simulink model "subsystem_enable_triggered"  (R2022b)
settings: Solver=VariableStepAuto  StartTime=0.0  StopTime=0.1  FixedStep=0.01  MaxStep=1e-3  RelTol=1e-3
settings Model: Creator=Dell  LastModifiedBy=Dell
settings OptimizationCC: DefaultParameterBehavior=Inlined  UseDivisionForNetSlopeComputation=on  GainParamInheritBuiltInType=on  UseFloatMulNetSlope=on  InlineInvariantSignals=on  PassReuseOutputArgsAs=Individual arguments  ZeroExternalMemoryAtStartup=off  ZeroInternalMemoryAtStartup=off  NoFixptDivByZeroProtection=on  EfficientFloat2IntCast=on  LifeSpan=1  OptimizeBlockOrder=speed  DifferentSizesBufferReuse=on  EfficientTunableParamExpr=on
settings DebuggingCC: ParameterTunabilityLossMsg=error
settings HardwareCC: ProdBitPerPointer=32  ProdBitPerSizeT=32  ProdBitPerPtrDiffT=32  ProdLargestAtomicInteger=Long  ProdLargestAtomicFloat=Double  ProdWordSize=32  ProdLongLongMode=on  ProdHWDeviceType=ARM Compatible->ARM Cortex-M
settings SFSimCC: MATLABDynamicMemAlloc=off
settings RTWCC: Description=Embedded Coder  SystemTargetFile=ert.tlc  TemplateMakefile=ert_default_tmf
settings CodeAppCC: ForceParamTrailComments=on  IgnoreCustomStorageClasses=off  OperatorAnnotations=on  SimulinkDataObjDesc=on  SFDataObjDesc=on  CustomSymbolStrGlobalVar=rt$N$M  CustomSymbolStrType=$N$M  CustomSymbolStrFcn=$N$M$F  CustomSymbolStrMacro=$N$M  InsertBlockDesc=on
settings ERTTargetCC: TargetLangStandard=C99 (ISO)  GenerateSampleERTMain=on  IncludeMdlTerminateFcn=off  CombineSignalStateStructs=on  SuppressErrorStatus=on  SupportAbsoluteTime=off  SupportComplex=off  InlinedParameterPlacement=NonHierarchical  ERTCustomFileTemplate=example_file_process.tlc  ERTFilePackagingFormat=CompactWithDataFile

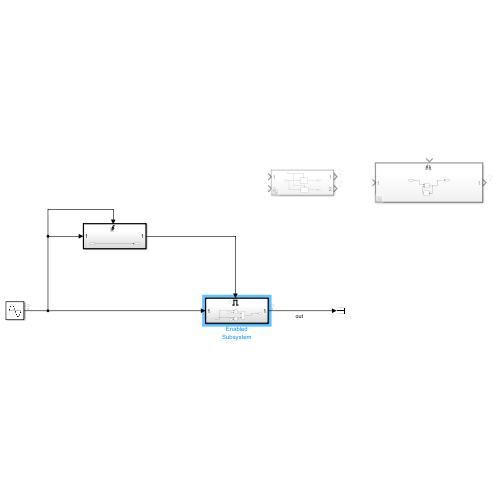
[thumbnail: Simulink's stored preview of the top-level diagram]
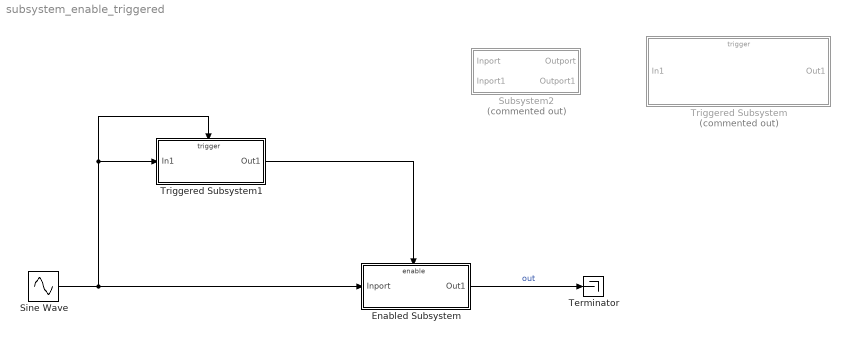
== system subsystem_enable_triggered ==
  Enabled Subsystem : Subsystem  TreatAsAtomicUnit=on
  Sine Wave : Sin  Amplitude=220  Frequency=2*pi*50  SampleTime=0
  Subsystem2 : Subsystem  Commented=on
  Terminator : Terminator
  Triggered Subsystem : Subsystem  Commented=on  TreatAsAtomicUnit=on
  Triggered Subsystem1 : Subsystem  TreatAsAtomicUnit=on
  wires:
  Enabled Subsystem/1(Out1) -> Terminator/1  "out"
  Sine Wave/1 -> Triggered Subsystem1/1(In1), Triggered Subsystem1/Trigger, Enabled Subsystem/1(Inport)
  Triggered Subsystem1/1(Out1) -> Enabled Subsystem/Enable

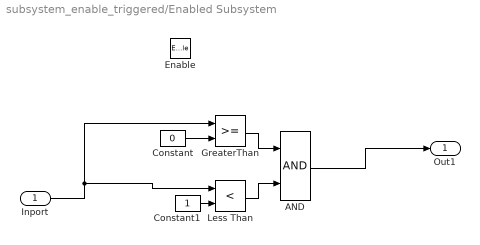
== system subsystem_enable_triggered/Enabled Subsystem ==
  Inport : Inport
  Enable : EnablePort
  AND : Logic  AllPortsSameDT=off  OutDataTypeStr=boolean
  Constant : Constant  Value=0
  Constant1 : Constant
  GreaterThan : RelationalOperator  OutDataTypeStr=boolean  RndMeth=Simplest  InputSameDT=off
  Less Than : RelationalOperator  Operator=<  OutDataTypeStr=boolean  RndMeth=Simplest  InputSameDT=off
  Out1 : Outport
  wires:
  Inport/1 -> GreaterThan/1, Less Than/1
  Constant1/1 -> Less Than/2
  Less Than/1 -> AND/2
  GreaterThan/1 -> AND/1
  Constant/1 -> GreaterThan/2
  AND/1 -> Out1/1

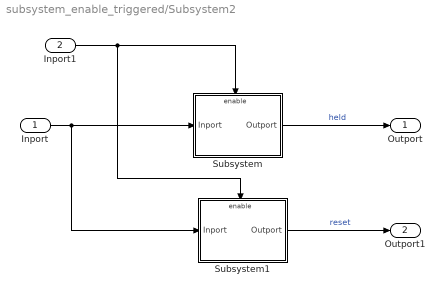
== system subsystem_enable_triggered/Subsystem2 ==
  Inport : Inport
  Inport1 : Inport  Port=2
  Subsystem : Subsystem
  Subsystem1 : Subsystem
  Outport : Outport
  Outport1 : Outport  Port=2
  wires:
  Subsystem/1(Outport) -> Outport/1  "held"
  Inport/1 -> Subsystem1/1(Inport), Subsystem/1(Inport)
  Subsystem1/1(Outport) -> Outport1/1  "reset"
  Inport1/1 -> Subsystem1/Enable, Subsystem/Enable

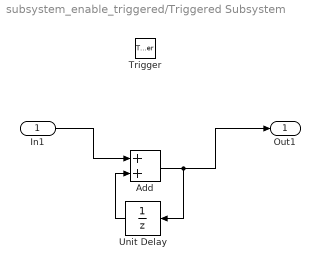
== system subsystem_enable_triggered/Triggered Subsystem ==
  In1 : Inport
  Trigger : TriggerPort  TriggerType=either  VariantControl=(inherit)
  Add : Sum
  Unit Delay : UnitDelay  SampleTime=-1  HasFrameUpgradeWarning=on
      settings: AttributesFormatString=InitialCondition=0
  Out1 : Outport
  wires:
  Unit Delay/1 -> Add/2
  In1/1 -> Add/1
  Add/1 -> Unit Delay/1, Out1/1

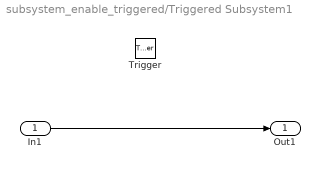
== system subsystem_enable_triggered/Triggered Subsystem1 ==
  In1 : Inport
  Trigger : TriggerPort  VariantControl=(inherit)
  Out1 : Outport
  wires:
  In1/1 -> Out1/1

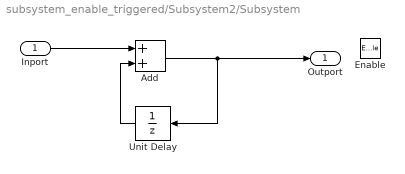
== system subsystem_enable_triggered/Subsystem2/Subsystem ==
  Inport : Inport
  Enable : EnablePort
  Add : Sum
  Unit Delay : UnitDelay  SampleTime=-1  HasFrameUpgradeWarning=on
      settings: AttributesFormatString=InitialCondition =0
  Outport : Outport
  wires:
  Add/1 -> Outport/1, Unit Delay/1
  Inport/1 -> Add/1
  Unit Delay/1 -> Add/2

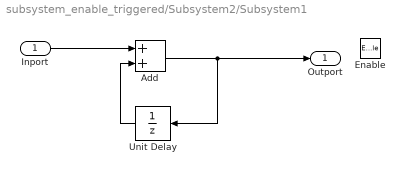
== system subsystem_enable_triggered/Subsystem2/Subsystem1 ==
  Inport : Inport
  Enable : EnablePort  StatesWhenEnabling=reset
  Add : Sum
  Unit Delay : UnitDelay  SampleTime=-1  HasFrameUpgradeWarning=on
      settings: AttributesFormatString=InitialCondition =0
  Outport : Outport
  wires:
  Unit Delay/1 -> Add/2
  Inport/1 -> Add/1
  Add/1 -> Unit Delay/1, Outport/1
